simulink model "GaitAlgorithm_arduino_V3_2024a"  (R2024b)
settings: Solver=FixedStepAuto  StartTime=0.0  StopTime=inf  RelTol=1e-3  EnableMultiTasking=on
undefined symbols (not defined in the file): DiscIntNeverNeededParam, f
libraries: simulink x16, mcp2515lib x13, matrix_library x6, arduinosensorlib x4, eeGeneralControl x4, arduinolib x2, instrumentlib x2
(part 1 of 2)
settings Model: ExtModeTrigDuration=2  Creator=82108  LastModifiedBy=admin
settings SolverCC: AutoInsertRateTranBlk=on
settings OptimizationCC: EnhancedBackFolding=on  PassReuseOutputArgsAs=Individual arguments  ZeroExternalMemoryAtStartup=off  ZeroInternalMemoryAtStartup=off  MaxStackSize=64  OptimizeBlockOrder=speed  DifferentSizesBufferReuse=on  OptimizationCustomize=off  EfficientTunableParamExpr=on
settings DebuggingCC: ParameterTunabilityLossMsg=error
settings HardwareCC: ProdBitPerInt=16  ProdBitPerPointer=16  ProdBitPerSizeT=16  ProdBitPerPtrDiffT=16  ProdLargestAtomicFloat=None  ProdWordSize=8  ProdHWDeviceType=Atmel->AVR  TargetBitPerPointer=64  TargetBitPerSizeT=64  TargetBitPerPtrDiffT=64  TargetLongLongMode=on  TargetIntDivRoundTo=Zero  TargetEndianess=LittleEndian  TargetWordSize=64  TargetHWDeviceType=Custom Processor->MATLAB Host Computer  ProdEqTarget=off
settings SFSimCC: MATLABDynamicMemAlloc=off
settings RTWCC: Description=Embedded Coder  SystemTargetFile=ert.tlc  HardwareBoard=Arduino Uno  TemplateMakefile=ert_default_tmf  Toolchain=Arduino AVR  BuildConfiguration=Faster Runs  GPUComputeCapability=3.5
settings CodeAppCC: ForceParamTrailComments=on  IgnoreCustomStorageClasses=off  OperatorAnnotations=on  SimulinkDataObjDesc=on  SFDataObjDesc=on  InsertBlockDesc=on
settings ERTTargetCC: SupportContinuousTime=on  SupportVariableSizeSignals=on  ExtModeTransport=3  ExtModeStaticAlloc=on  ExtModeAutomaticAllocSize=off  ExtModeStaticAllocSize=250  ExtModeMexFile=ext_xcp  ExtModeIntrfLevel=Level2 - Open  InlinedParameterPlacement=Hierarchical  DynamicArrayContainerType=coder::array

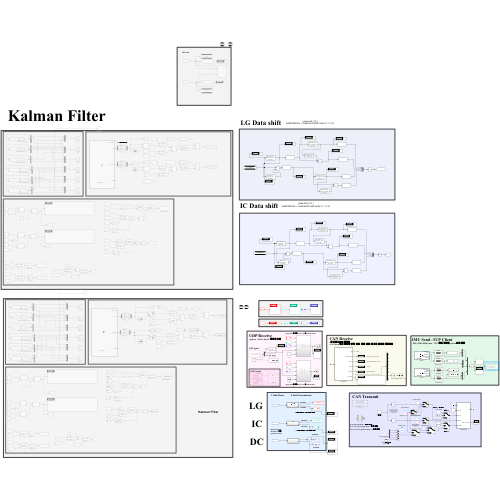
[thumbnail: Simulink's stored preview of the top-level diagram]
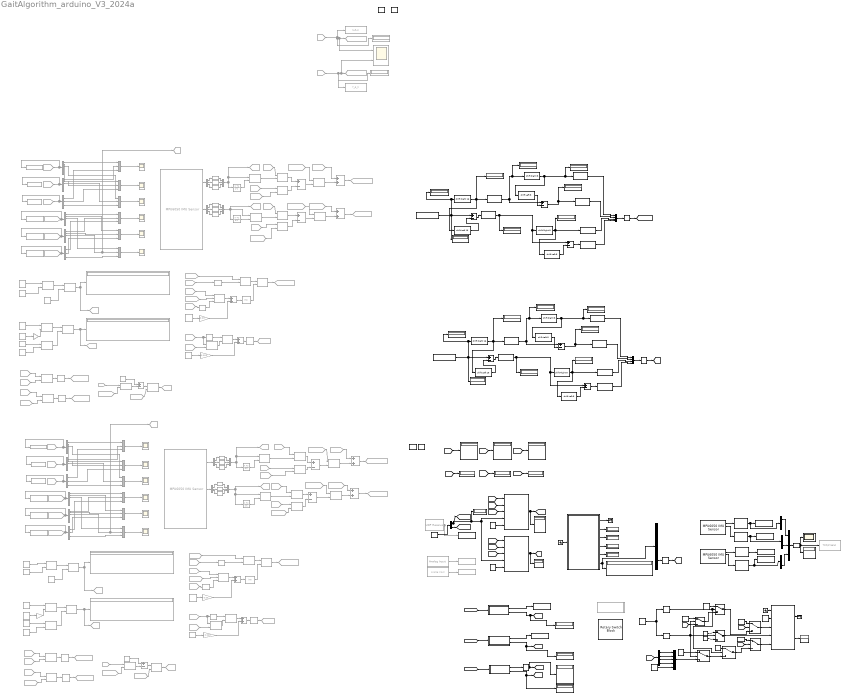
== system GaitAlgorithm_arduino_V3_2024a ==
  note: data 전달받았는지 확인
  note: gait phase에 따른 DC, IC, LG 의 position value
  note: LG Data shift
  note: [ data shift 과정 ]
      | 0xABCDEFGH -> 0xAB 0xCD 0xEF 0xGH 로 나눠줌
  note: position
  note: Kalman Filter
  note: IMU data
  note: Kalman Filter
  note: bias 로 영점 조절
  note: DC
  note: MobileNetHED- Double3D 기반
      | gait phase label
  note: 16진수 데이터 ID로 나눠서 전송
  note: id value
  note: Gait Phase
  note: 2. Data Transmission
  note: 16진수 데이터 ID로 나눠서 전송
  note: id value
  note: position
  note: LG
  note: IC
  note: position
  note: id value
  note: CAN Receive
      | :모터에 나오는 데이터
      | :CAN data에서 모터의 위치, 속도, 전류, 온도 등 모터 정보를 제공받음
  note: gait phase에 따른 DC, IC, LG 의 CAN id value
  note: UDP signal
  note: EMG signal
  note: extended version인지 확인
  note: id 확인
  note: data length 확인
  note: 온도 255 degree 넘으면 중지
  note: etc
  note: etc
  note: IC Data shift
  note: IMU Send -TCP Client
      | :IMU (MPU6050) data - TCP 통신 이용해 python으로 전달
  note: UDP Receive
      | :python - label1, label2 데이터 수신
  note: [ data shift 과정 ]
      | 0xABCDEFGH -> 0xAB 0xCD 0xEF 0xGH 로 나눠줌
  note: 모드
  note: motor position value
  note: D (0): Driving mode - 운용 모드
      | Z (1): Zeroing (origin) mode - 영점 조절
      | TZ (2): To Zero position mode - 0으로 복귀
  note: 틀리면 0 / 맞으면 1
      | - driving mode: 00
      | - zeroing mode: 01
      | - to zero: 10
  note: driving mode : id
  note: driving mode
      | & to zero mode : DLC
  note: 온도 limit
  note: to zero mode : data
  note: 온도 limit
  note: zeroing mode : DLC
  note: 온도가 limit 초과할 시,
      | to zero mode
  note: CAN Transmit
  note: to zero mode : id
  note: shape 맞추기 위한 dummy 값
  note: zeroing mode : id
  note: zeroing mode :
      | data
  Acc_x : Scope  Commented=on
  Acc_x1 : Scope  Commented=on
  Acc_y : Scope  Commented=on
  Acc_y1 : Scope  Commented=on
  Acc_z : Scope  Commented=on
  Acc_z1 : Scope  Commented=on
  Add{,1,6,9..10,13..15} (8 alike) : Sum  Commented=on
  Add{5,7..8,11..12,16} (6 alike) : Sum  Commented=on  Inputs=+-
  Add{2..4,17..19} (6 alike) : Sum  Inputs=+-
  Analog Input : arduinolib/Analog Input  Commented=on  pinNumber=0  ReadResultsOnly=off  ConversionTriggerSource=Software  ExternalTriggerType=uint32( 0 )  OutputDataType=uint16  EnableConversionCompleteNotify=off  EnableOuputStatus=off  SampleTime=0.01  blockPlatform=arduino
      settings: SourceProductName=Common
  Analog Input1 : arduinolib/Analog Input  Commented=on  pinNumber=1  ReadResultsOnly=off  ConversionTriggerSource=Software  ExternalTriggerType=uint32( 0 )  OutputDataType=uint16  EnableConversionCompleteNotify=off  EnableOuputStatus=off  SampleTime=0.01  blockPlatform=arduino
      settings: SourceProductName=Common
  Bias{,1..11} (12 alike) : Bias  Commented=on  SaturateOnIntegerOverflow=off
  CANbegin : Subsystem  Commented=on  TreatAsAtomicUnit=on  mask{TargetHardware=Arduino, Oscillator=8, CANSpeed=1000, CSpin=10}
      mask prompts: TargetHardware "Target Hardware"; Oscillator "Oscillator frequency(MHz)"; CANSpeed "CAN speed(kHz)"; CSpin "Chip Select Pin"
      mask init:
      | % Get this mask's handle
      | maskObj = Simulink.Mask.get(gcb);
      | 
      | % Get the selected value from mask parameter's option
      | str_TargetHard = char(maskObj.Parameters(1).TypeOptions(TargetHardware));
      | str_Osc = char(maskObj.Parameters(2).TypeOptions(Oscillator));
      | str_CANSpeed = char(maskObj.Parameters(3).TypeOptions(CANSpeed));
      | 
      | % Set Icon
      | str1 = sprintf('%s(Model)',str_TargetHard);
      | str2 = sprintf('Oscillator: %s(MHz)',str_Osc);
      | str3 = sprintf('CAN Bus Speed: %s(kHz)',str_CANSpeed);
      | str4 = sprintf('Chip Select pin: %d',CSpin);
      | 
      | % Set the values of Variant Subsystem
      | switch str_TargetHard
      |     case 'Arduino'
      |         str = [str1,'\n',str2,'\n',str3,'\n',str4];
      |         evalin('base',sprintf('CSpin = %d;',CSpin));        
      |         evalin('base','Hardware = 1;');
      |     case 'Raspberry Pi'
      |         str = [str1,'\n',str2,'\n',str3];
      |         evalin('base',sprintf('clear CSpin',CSpin));           
      |         evalin('base','Hardware = 2;');     
      | end  
      | 
      | % Get the CAN Configuration register's value from mask parameter's option
      | if str_Osc == '8' %[MHz]
      |     switch str_CANSpeed
      |         case '1000'
      |             BPR = 0; PHSEG1 = 0; PRSEG = 0; PHSEG2 = 0;
      |         case '500'
      |             BPR = 0; PHSEG1 = 2; PRSEG = 0; PHSEG2 = 2;
      |         case '250'
      |             BPR = 0; PHSEG1 = 6; PRSEG = 0; PHSEG2 = 6;
      |         case '125'
      |             BPR = 1; PHSEG1 = 6; PRSEG = 1; PHSEG2 = 5;
      |         case '100'
      |             BPR = 1; PHSEG1 = 7; PRSEG = 2; PHSEG2 = 7;
      |         case '83.3'
      |             BPR = 1; PHSEG1 = 7; PRSEG = 6; PHSEG2 = 7;
      |         case '62.5'
      |             BPR = 3; PHSEG1 = 6; PRSEG = 0; PHSEG2 = 6;
      |         case '50'
      |             BPR = 3; PHSEG1 = 7; PRSEG = 2; PHSEG2 = 7;
      |         case '33.3'
      |             BPR = 4; PHSEG1 = 7; PRSEG = 6; PHSEG2 = 7;
      |     end            
      | elseif str_Osc == '16' %[MHz]
      |     switch str_CANSpeed  
      |         case '1000'
      |             BPR = 0; PHSEG1 = 2; PRSEG = 0; PHSEG2 = 2;
      |         case '500'
      |             BPR = 0; PHSEG1 = 6; PRSEG = 0; PHSEG2 = 6;
      |         case '250'
      |             BPR = 1; PHSEG1 = 6; PRSEG = 1; PHSEG2 = 5;        
      |         case '125'
      |             BPR = 3; PHSEG1 = 6; PRSEG = 0; PHSEG2 = 6;
      |         case '100'
      |             BPR = 3; PHSEG1 = 7; PRSEG = 2; PHSEG2 = 7;
      |         case '83.3'
      |             BPR = 3; PHSEG1 = 7; PRSEG = 6; PHSEG2 = 7;
      |         case '62.5'
      |             BPR = 7; PHSEG1 = 6; PRSEG = 0; PHSEG2 = 6;
      |         case '50'
      |             BPR = 7; PHSEG1 = 7; PRSEG = 2; PHSEG2 = 7;
      |         case '33.3'
      |             BPR = 9; PHSEG1 = 7; PRSEG = 6; PHSEG2 = 7;        
      |     end   
      | end
      | % Set the CAN Configuration register's value
      | address2A = BPR;          % bit7-6 :SJW, bit5-0: BPR
      | address29 = 192 ...       % bit7: BTLMODE = 1, bit6:SAM = 1
      |             + 8*PHSEG1 ...% bit5-3: PHSEG1
      |             +PRSEG;       % bit2-0: PRSEG
      | address28 = 128 ...       % bit7: SOF = 1, bit6:WAKFIL = 0
      |             + PHSEG2;     % bit5-3: 0, bit2-0: PHSEG2
      settings: RTWSystemCode=Nonreusable function
      mask TypeOptions TargetHardware: Arduino | Raspberry Pi
      mask Callback TargetHardware:
      | if(strcmp(get_param(gcb,'TargetHardware'),'Arduino'))
      |     set_param(gcb,'MaskVisibilities',{'on','on','on','on'})
      | else
      |     set_param(gcb,'MaskVisibilities',{'on','on','on','off'})
      | end
      mask TypeOptions Oscillator: 8 | 16
      mask TypeOptions CANSpeed: 1000 | 500 | 250 | 125 | 100 | 83.3 | 62.5 | 50 | 33.3
      mask DialogControl DescGroupVar Prompt: Description
      mask DialogControl DescTextVar Prompt: This block must be executed only once when beginning CAN communication because MCP2515’s register needs to be configured. And the frequency of oscillator for MCP2515 is also needed because it effects to the setting parameters of MCP2515's register.
      mask Display: disp(str)
  CANreceive : Subsystem  TreatAsAtomicUnit=on
      mask DialogControl DescGroupVar Prompt: Description
      mask DialogControl DescTextVar Prompt: CANreceive outputs CAN data by converting MCP2515 RX buffer register’s values. In/Out ports are no use because they are used for controlling the execution order. CAN_Received outputs 1(CAN received) or -1( No message).
  CANtransmit : Subsystem  TreatAsAtomicUnit=on
      mask DialogControl DescGroupVar Prompt: Description
      mask DialogControl DescTextVar Prompt: CANtransmit inputs CAN data by converting MCP2515 TX buffer register’s values. In/Out ports are no use because they are used for controlling the execution order. CAN_Transmitted outputs 1(Success) or 2(Fail).
  Compare To Constant7 : simulink/Logic and Bit Operations/Compare To Constant  relop===  const=1  OutDataTypeStr=boolean
  Compare To Constant8 : simulink/Logic and Bit Operations/Compare To Constant  relop===  const=2  OutDataTypeStr=boolean
  Compare To Constant9 : simulink/Logic and Bit Operations/Compare To Constant  relop=>=  const=0xff  OutDataTypeStr=boolean
  Constant : Constant  Value=[0 0 0 0]  OutDataTypeStr=uint8
  Constant1 : Constant  OutDataTypeStr=uint8
  Constant10 : Constant  Commented=on  Value=[0 0 0; 0 0 0; 0 0 0]  SampleTime=-1
  Constant11 : Constant  Commented=on  Value=[0 0 0; 0 0 0; 0 0 0]
  Constant12 : Constant  Commented=on  Value=[0 0 0 0 0 0; 0 0 0 0 0 0; 0 0 0 0 0 0]
  Constant13 : Constant  Commented=on  Value=[0 0 0; 0 0 0; 0 0 0]
  Constant14 : Constant  Value=0x168  OutDataTypeStr=uint16
  Constant15 : Constant  Value=[0x00 0x00 0x07 0xd0 ]  OutDataTypeStr=uint16
  Constant2 : Constant  Value=[1,1]
  Constant21 : Constant  Value=0x468
  Constant22 : Constant  Value=[0 0 0 0 0 0 0 0 ]  OutDataTypeStr=uint8
  Constant23 : Constant  Value=0x468
  Constant24 : Constant  Value=[0 0 0 0 0 0 0 0 ]  OutDataTypeStr=uint8
  Constant25 : Constant
  Constant3 : Constant  Value=4  OutDataTypeStr=uint8
  Constant5 : Constant  Value=0x568
  Constant6 : Constant  OutDataTypeStr=uint8
  Constant7 : Constant  Value=[0x01 0 0 0 0 0 0 0]  OutDataTypeStr=uint8
  Constant8 : Constant  Commented=on  Value=[0 0 0; 0 0 0; 0 0 0]
  Constant9 : Constant  Commented=on  Value=[0 0 0 0 0 0; 0 0 0 0 0 0; 0 0 0 0 0 0]  SampleTime=-1
  Data Store Memory : DataStoreMemory  DataStoreName=T_G_Z  WriteAfterWriteMsg=warning  ShowAdditionalParam=off
  Data Store Memory1 : DataStoreMemory  DataStoreName=S_G_Z  WriteAfterWriteMsg=warning  ShowAdditionalParam=off
  Data Store Memory2 : DataStoreMemory  DataStoreName=LG_position  WriteAfterWriteMsg=warning  ShowAdditionalParam=off
  Data Store Memory4 : DataStoreMemory  DataStoreName=IC_position  WriteAfterWriteMsg=warning  ShowAdditionalParam=off
  Data Store Read : DataStoreRead  DataStoreName=LG_position  IndexOptions=Index vector (dialog)  Indices=1  OutputSizes=1
  Data Store Read3 : DataStoreRead  DataStoreName=IC_position  IndexOptions=Index vector (dialog)  Indices=1  OutputSizes=1
  Data Store Write : DataStoreWrite  Commented=on  DataStoreName=T_G_Z  DataStoreElements=T_G_Z  IndexOptions=Index vector (dialog)  Indices=1  OutputSizes=1
  Data Store Write1 : DataStoreWrite  Commented=on  DataStoreName=S_G_Z  DataStoreElements=S_G_Z  IndexOptions=Index vector (dialog)  Indices=1  OutputSizes=1
  Data Store Write2 : DataStoreWrite  DataStoreName=LG_position  IndexOptions=Index vector (dialog)  Indices=1  OutputSizes=1
  Data Store Write3 : DataStoreWrite  DataStoreName=IC_position  IndexOptions=Index vector (dialog)  Indices=1  OutputSizes=1
  Data Type Conversion{1..2,10..11} (4 alike) : DataTypeConversion  OutDataTypeStr=uint16  SaturateOnIntegerOverflow=off  RndMeth=Floor
  Data Type Conversion{6..7,9,12} (4 alike) : DataTypeConversion  OutDataTypeStr=uint8  SaturateOnIntegerOverflow=off  RndMeth=Floor
  Data Type Conversion{3..5,8} (4 alike) : DataTypeConversion  OutDataTypeStr=uint8  RndMeth=Floor
  Delay1 : Delay  Commented=on  DelayLength=1
  Delay2 : Delay  Commented=on  DelayLength=1
  Delay_acc : Delay  Commented=on  DelayLength=1  InitialCondition=[0; 0; 0; 0; 0;0]
  Delay_acc1 : Delay  Commented=on  DelayLength=1  InitialCondition=[0; 0; 0; 0; 0;0]
  Delay_gyro : Delay  Commented=on  DelayLength=1  InitialCondition=[0; 0; 0; 0; 0;0]
  Delay_gyro1 : Delay  Commented=on  DelayLength=1  InitialCondition=[0; 0; 0; 0; 0;0]
  Demux : Demux  Outputs=8
  Demux1 : Demux  Outputs=3
  Demux{3..4,6..7,9..10,16,18} (8 alike) : Demux  Commented=on  Outputs=6
  Demux{5,8,11..15,17} (8 alike) : Demux  Commented=on  Outputs=3
  Demux19 : Demux  Outputs=3
  Demux2 : Demux
  Demux20 : Demux  Outputs=3
  Demux22 : Demux  Outputs=2
  Discrete-Time Integrator{,1..3} (4 alike) : DiscreteIntegrator  Commented=on  SampleTime=-1  ICPrevOutput=DiscIntNeverNeededParam  ICPrevScaledInput=DiscIntNeverNeededParam
  Display{,1,7,9..41} (36 alike) : Display
      Display11 settings: Format=hex (Stored Integer)
      Display12 settings: Format=hex (Stored Integer)
      Display13 settings: Format=hex (Stored Integer)
      Display14 settings: Format=hex (Stored Integer)
      Display15 settings: Format=hex (Stored Integer)
      Display16 settings: Format=hex (Stored Integer)
      Display17 settings: Format=hex (Stored Integer)
      Display18 settings: Format=hex (Stored Integer)
      Display19 settings: Format=hex (Stored Integer)
      Display20 settings: Format=hex (Stored Integer)
      Display21 settings: Format=hex (Stored Integer)
      Display22 settings: Format=hex (Stored Integer)
      Display23 settings: Format=hex (Stored Integer)
      Display24 settings: Format=hex (Stored Integer)
      Display28 settings: Format=hex (Stored Integer)
      Display30 settings: Format=hex (Stored Integer)
      Display32 settings: Format=hex (Stored Integer)
      Display7 settings: Format=hex (Stored Integer)
  Display{2..6,8} (6 alike) : Display  Commented=on
  Enabled Subsystem1 : Subsystem  TreatAsAtomicUnit=on
  Enabled Subsystem3 : Subsystem  TreatAsAtomicUnit=on
  Enabled Subsystem4 : Subsystem  TreatAsAtomicUnit=on
  Estimated_Data_acc : From  Commented=on  GotoTag=x_hat
  Estimated_Data_acc1 : From  Commented=on  GotoTag=x_hat_2
  Estimated_Data_gyro : From  Commented=on  GotoTag=AR_x_hat
  Estimated_Data_gyro1 : From  Commented=on  GotoTag=AR_x_hat_2
  From1 : From  Commented=on  GotoTag=C_Phi
  From10 : From  Commented=on  GotoTag=AR_x_bar
  From12 : From  Commented=on  GotoTag=x_hat
  From{3,9,13,18,48..51} (8 alike) : From  Commented=on  GotoTag=H
  From14 : From  Commented=on  GotoTag=x_bar
  From15 : From  Commented=on  GotoTag=kalmangain
  From16 : From  Commented=on  GotoTag=x_bar
  From17 : From  Commented=on  GotoTag=kalmangain
  From19 : From  Commented=on  GotoTag=cov_bar
  From2 : From  Commented=on  GotoTag=cov
  From20 : From  Commented=on  GotoTag=C_Phi_2
  From21 : From  Commented=on  GotoTag=cov_2
  From22 : From  Commented=on  GotoTag=AR_x_bar_2
  From23 : From  Commented=on  GotoTag=kalmangain
  From24 : From  Commented=on  GotoTag=AR_x_bar
  From25 : From  Commented=on  GotoTag=C_Phi
  From26 : From  Commented=on  GotoTag=AR_x_hat
  From{27,29,34,43..47} (8 alike) : From  Commented=on  GotoTag=H_2
  From28 : From  Commented=on  GotoTag=x_hat_2
  From30 : From  Commented=on  GotoTag=x_bar_2
  From31 : From  Commented=on  GotoTag=kalmangain_2
  From32 : From  Commented=on  GotoTag=x_bar_2
  From33 : From  Commented=on  GotoTag=kalmangain_2
  From35 : From  Commented=on  GotoTag=cov_bar_2
  From36 : From  Commented=on  GotoTag=C_Phi_2
  From37 : From  Commented=on  GotoTag=kalmangain_2
  From38 : From  Commented=on  GotoTag=AR_x_bar_2
  From39 : From  Commented=on  GotoTag=C_Phi_2
  From4 : From  Commented=on  GotoTag=C_Phi
  From40 : From  Commented=on  GotoTag=AR_x_hat_2
  From41 : From  Commented=on  GotoTag=cov_bar_2
  From42 : From  Commented=on  GotoTag=cov_bar_2
  From5 : From  Commented=on  GotoTag=cov_bar
  From52 : From  Commented=on  GotoTag=TGZ
  From53 : From  Commented=on  GotoTag=SGZ
  From6 : From  Commented=on  GotoTag=cov_bar
  Gain : Gain  Commented=on  Gain=-0.01
  Gain1 : Gain  Commented=on  Gain=-0.01
  Goto : Goto  Commented=on  GotoTag=thigh_gyro_z
  Goto1 : Goto  Commented=on  GotoTag=C_Phi
  Goto10 : Goto  Commented=on  GotoTag=AR_x_bar
  Goto11 : Goto  Commented=on  GotoTag=x_hat_2
  Goto12 : Goto  Commented=on  GotoTag=AR_x_bar_2
  Goto13 : Goto  Commented=on  GotoTag=x_bar_2
  Goto14 : Goto  Commented=on  GotoTag=cov_bar_2
  Goto15 : Goto  Commented=on  GotoTag=H_2
  Goto16 : Goto  Commented=on  GotoTag=cov_2
  Goto17 : Goto  Commented=on  GotoTag=x_2
  Goto18 : Goto  Commented=on  GotoTag=AR_x_hat_2
  Goto19 : Goto  Commented=on  GotoTag=AR_x_2
  Goto2 : Goto  Commented=on  GotoTag=x_hat
  Goto20 : Goto  Commented=on  GotoTag=cov
  Goto21 : Goto  Commented=on  GotoTag=x
  Goto22 : Goto  Commented=on  GotoTag=AR_x_hat
  Goto23 : Goto  Commented=on  GotoTag=AR_x
  Goto24 : Goto  Commented=on  GotoTag=SGZ
  Goto25 : Goto  Commented=on  GotoTag=TGZ
  Goto4 : Goto  Commented=on  GotoTag=x_bar
  Goto6 : Goto  Commented=on  GotoTag=shank_gyro_z
  Goto7 : Goto  Commented=on  GotoTag=cov_bar
  Goto8 : Goto  Commented=on  GotoTag=C_Phi_2
  Goto9 : Goto  Commented=on  GotoTag=H
  Ground : Ground
  Ground1 : Ground
  Gyro_x : Scope  Commented=on
  Gyro_x1 : Scope  Commented=on
  Gyro_y : Scope  Commented=on
  Gyro_y1 : Scope  Commented=on
  Gyro_z : Scope  Commented=on
  Gyro_z1 : Scope  Commented=on
  IdentityMatrix{,1..2,4,7..9,11} (8 alike) : IdentityMatrix  Commented=on  OutputDimensions=3  SampleTime=-1
  IdentityMatrix{3,5..6,10,12..13} (6 alike) : IdentityMatrix  Commented=on  OutputDimensions=6  SampleTime=-1
  Kalman_Gain : Goto  Commented=on  GotoTag=kalmangain
  Kalman_Gain1 : Goto  Commented=on  GotoTag=kalmangain_2
  MPU6050 IMU Sensor : arduinosensorlib/MPU6050 IMU Sensor  Commented=on  I2CModule=0  SlaveAddress=0x68  Accel=on  AngularRate=on  Temperature=off  Status=on  Timestamp=off  EulerAngles=off  Quat=off  AccelRange=2G  GyroRange=250 dps  DmpOdr=200 Hz  Dlpf=Accelerometer: 184Hz, Gyroscope: 188Hz  spf=1  SampleTime=0.01  QueueSizeFactor=1
      settings: SourceProductName=Sensors
  MPU6050 IMU Sensor1 : arduinosensorlib/MPU6050 IMU Sensor  Commented=on  I2CModule=0  SlaveAddress=0x69  Accel=on  AngularRate=on  Temperature=off  Status=on  Timestamp=off  EulerAngles=off  Quat=off  AccelRange=2G  GyroRange=250 dps  DmpOdr=200 Hz  Dlpf=Accelerometer: 184Hz, Gyroscope: 188Hz  spf=1  SampleTime=0.01  QueueSizeFactor=1
      settings: SourceProductName=Sensors
  Matrix Concatenate{,1,4,7..8,11} (6 alike) : Concatenate  Commented=on  Mode=Multidimensional array  ConcatenateDimension=2
  Matrix Concatenate{2..3,5..6,9..10,12..13} (8 alike) : Concatenate  Commented=on  Mode=Multidimensional array
  Matrix Divide : Product  Commented=on  Inputs=/  Multiplication=Matrix(*)
  Matrix Divide1 : Product  Commented=on  Inputs=/  Multiplication=Matrix(*)
  Matrix Multiply{,1..3,5..23,25..29} (28 alike) : Product  Commented=on  Multiplication=Matrix(*)
  Matrix Multiply24 : Product  Commented=on  Inputs=3  Multiplication=Matrix(*)
  Matrix Multiply4 : Product  Commented=on  Inputs=3  Multiplication=Matrix(*)
  Measurement_Data_acc : From  Commented=on  GotoTag=x
  Measurement_Data_acc1 : From  Commented=on  GotoTag=x_2
  Measurement_Data_gyro : From  Commented=on  GotoTag=AR_x
  Measurement_Data_gyro1 : From  Commented=on  GotoTag=AR_x_2
  Mux{,1..15} (16 alike) : Mux  Commented=on  Inputs=3
  Mux16 : Mux  Inputs=3
  Predicted_Data_acc : From  Commented=on  GotoTag=x_bar
  Predicted_Data_acc1 : From  Commented=on  GotoTag=x_bar_2
  Predicted_Data_gyro : From  Commented=on  GotoTag=AR_x_bar
  Predicted_Data_gyro1 : From  Commented=on  GotoTag=AR_x_bar_2
  Reshape1 : Reshape
  Reshape2 : Reshape
  Reshape3 : Reshape
  Reshape4 : Reshape  OutputDimensionality=Customize  OutputDimensions=[3,1]
  Rotary Switch : RotarySwitchBlock
      settings: Values={{'D', 'Z', 'TZ'}, [0 1 2]}
  Scope1 : Scope  Commented=on  NumInputPorts=2
  Scope2 : Scope
  Shift Arithmetic{1,7,10..11} (4 alike) : ArithShift  BitShiftNumber=8  BitShiftDirection=Right
  Shift Arithmetic13 : ArithShift  BitShiftNumber=16  BitShiftDirection=Right
  Shift Arithmetic{2,4,6,9} (4 alike) : ArithShift  BitShiftNumber=8  BitShiftDirection=Left
  Shift Arithmetic3 : ArithShift  BitShiftNumber=16  BitShiftDirection=Left
  Shift Arithmetic5 : ArithShift  BitShiftNumber=16  BitShiftDirection=Right
  Shift Arithmetic8 : ArithShift  BitShiftNumber=16  BitShiftDirection=Left
  Subsystem : Subsystem
  Subsystem1 : Subsystem
  Switch{,1..4,11..12} (7 alike) : Switch  Criteria=u2 > Threshold  SaturateOnIntegerOverflow=off  InputSameDT=off
  TCP/IP Send2 : instrumentlib/TCP//IP Send  Commented=on  Host=172.16.1.77  Port=5550  ByteOrder=little-endian  EnableBlockingMode=on  Timeout=10  TransferDelay=off  SimulateUsing=Interpreted execution
  Terminator : Terminator
  Terminator1 : Terminator
  To Workspace : ToWorkspace  Commented=on  VariableName=predicted_acc  SaveFormat=Timeseries  SampleTime=-1
  To Workspace1 : ToWorkspace  Commented=on  VariableName=measured_acc  SaveFormat=Timeseries  SampleTime=-1
  To Workspace10 : ToWorkspace  Commented=on  VariableName=estimated_gyro_shank  SaveFormat=Timeseries  SampleTime=-1
  To Workspace11 : ToWorkspace  Commented=on  VariableName=measured_gyro_shank  SaveFormat=Timeseries  SampleTime=-1
  To Workspace12 : ToWorkspace  VariableName=predicted  SaveFormat=Timeseries  SampleTime=-1
  To Workspace13 : ToWorkspace  Commented=on  VariableName=emg0  SaveFormat=Timeseries  SampleTime=-1
  To Workspace14 : ToWorkspace  Commented=on  VariableName=emg1  SaveFormat=Timeseries  SampleTime=-1
  To Workspace15 : ToWorkspace  VariableName=shank_acc  SaveFormat=Timeseries  SampleTime=0.01
  To Workspace16 : ToWorkspace  VariableName=shank_gyro  SaveFormat=Timeseries  SampleTime=0.01
  To Workspace17 : ToWorkspace  VariableName=thigh_acc  SaveFormat=Timeseries  SampleTime=-1
  To Workspace18 : ToWorkspace  VariableName=thigh_gyro  SaveFormat=Timeseries  SampleTime=-1
  To Workspace2 : ToWorkspace  Commented=on  VariableName=estimated_acc  SaveFormat=Timeseries  SampleTime=-1
  To Workspace3 : ToWorkspace  Commented=on  VariableName=predicted_gyro  SaveFormat=Timeseries  SampleTime=-1
  To Workspace4 : ToWorkspace  Commented=on  VariableName=estimated_gyro  SaveFormat=Timeseries  SampleTime=-1
  To Workspace5 : ToWorkspace  Commented=on  VariableName=measured_gyro  SaveFormat=Timeseries  SampleTime=-1
  To Workspace6 : ToWorkspace  Commented=on  VariableName=predicted_acc_shank  SaveFormat=Timeseries  SampleTime=-1
  To Workspace7 : ToWorkspace  Commented=on  VariableName=measured_acc_shank  SaveFormat=Timeseries  SampleTime=-1
  To Workspace8 : ToWorkspace  Commented=on  VariableName=estimated_acc_shank  SaveFormat=Timeseries  SampleTime=-1
  To Workspace9 : ToWorkspace  Commented=on  VariableName=predicted_gyro_shank  SaveFormat=Timeseries  SampleTime=-1
  Transpose{,1..5} (6 alike) : matrix_library/Transpose  Commented=on
  UDP Receive : instrumentlib/UDP Receive  Commented=on  LocalAddress=172.16.1.77  LocalPort=8888  EnablePortSharing=off  Host=localhost  Port=9090  GetLatestData=off  DataSize=[ 2, 1 ]  DataType=uint8  ASCIIFormatting=%f,  Terminator=LF  CustomTerminator=10  ByteOrder=big-endian  EnableBlockingMode=on  Timeout=10  SampleTime=0.1  SimulateUsing=Interpreted execution
  Vector Concatenate1 : Concatenate  NumInputs=4  ConcatenateDimension=2
  Vector Concatenate2 : Concatenate  NumInputs=4  ConcatenateDimension=2
  Vector Concatenate3 : Concatenate  NumInputs=5
  sensor noise : Gain  Commented=on  Gain=0.03
  sensor noise1 : Gain  Commented=on  Gain=0.03
  shank1 : arduinosensorlib/MPU6050 IMU Sensor  I2CModule=0  SlaveAddress=0x68  Accel=on  AngularRate=on  Temperature=on  Status=on  Timestamp=off  EulerAngles=off  Quat=off  AccelRange=2G  GyroRange=250 dps  DmpOdr=200 Hz  Dlpf=Accelerometer: 184Hz, Gyroscope: 188Hz  spf=1  SampleTime=0.01  QueueSizeFactor=1
      settings: SourceProductName=Sensors
  shank_acc1 : eeGeneralControl/Low-Pass Filter (Discrete or Continuous)  K=1  T=0.029  B=inf  A=-inf  init_option=Inherited from block input  x0=0  Ts=0.01
  shank_gyro1 : eeGeneralControl/Low-Pass Filter (Discrete or Continuous)  K=1  T=0.029  B=inf  A=-inf  init_option=Inherited from block input  x0=0  Ts=-1
  system noise : Gain  Commented=on  Gain=0.005
  system noise1 : Gain  Commented=on  Gain=0.005
  thigh1 : arduinosensorlib/MPU6050 IMU Sensor  I2CModule=0  SlaveAddress=0x69  Accel=on  AngularRate=on  Temperature=on  Status=on  Timestamp=off  EulerAngles=off  Quat=off  AccelRange=2G  GyroRange=250 dps  DmpOdr=200 Hz  Dlpf=Accelerometer: 184Hz, Gyroscope: 188Hz  spf=1  SampleTime=0.01  QueueSizeFactor=1
      settings: SourceProductName=Sensors
  thigh_acc1 : eeGeneralControl/Low-Pass Filter (Discrete or Continuous)  K=1  T=0.029  B=inf  A=-inf  init_option=Inherited from block input  x0=0  Ts=-1
  thigh_gyro1 : eeGeneralControl/Low-Pass Filter (Discrete or Continuous)  K=1  T=0.029  B=inf  A=-inf  init_option=Inherited from block input  x0=0  Ts=-1
  wires:
  From52/1 -> Data Store Write/1, Display3/1, Scope1/2, Goto/1
  From53/1 -> Display2/1, Scope1/1, Goto6/1, Data Store Write1/1
  Add16/1 -> Matrix Multiply28/2
  Mux3/1 -> Gyro_x/1
  From24/1 -> Add9/1
  From10/1 -> Matrix Multiply12/2
  Demux6/2 -> Mux4/1
  Demux8/2 -> Mux4/3
  Demux7/3 -> Goto24/1, Mux5/2
  Measurement_Data_gyro/1 -> To Workspace5/1, Demux8/1
  Matrix Multiply13/1 -> Add9/2
  Transpose3/1 -> Matrix Multiply22/1
  From23/1 -> Matrix Multiply13/1
  Demux5/3 -> Mux2/3
  Estimated_Data_acc/1 -> To Workspace2/1, Demux4/1
  Demux3/3 -> Mux2/1
  Matrix Multiply11/1 -> Add8/1
  Demux5/2 -> Mux1/3
  Matrix Multiply9/1 -> Add7/2
  Add1/1 -> Matrix Divide/1
  Transpose2/1 -> Matrix Multiply4/3
  Matrix Multiply3/1 -> Matrix Multiply5/1
  From9/1 -> Transpose1/1
  From3/1 -> Matrix Multiply/1
  From13/1 -> Matrix Multiply7/1
  From12/1 -> Matrix Multiply6/2
  Transpose1/1 -> Matrix Multiply3/2
  Matrix Divide/1 -> Matrix Multiply5/2
  From5/1 -> Matrix Multiply3/1
  Delay_acc/1 -> Goto4/1
  Matrix Multiply5/1 -> Kalman_Gain/1
  Matrix Concatenate1/1 -> Matrix Concatenate2/2
  From48/1 -> Transpose2/1
  IdentityMatrix3/1 -> system noise/1
  Gain/1 -> Matrix Concatenate/2
  Matrix Concatenate4/1 -> Matrix Concatenate6/1
  From2/1 -> Matrix Multiply1/2
  Constant10/1 -> Matrix Concatenate4/2
  Delay1/1 -> Goto7/1
  Matrix Concatenate3/1 -> Matrix Multiply/2
  From4/1 -> Matrix Multiply1/1, Transpose/1
  Predicted_Data_acc/1 -> Demux3/1, To Workspace/1
  Matrix Concatenate2/1 -> Goto1/1, Display5/1
  Predicted_Data_gyro/1 -> To Workspace3/1, Demux6/1
  Matrix Concatenate6/1 -> Goto9/1, Display4/1
  Mux7/1 -> Acc_y1/1
  system noise/1 -> Add/2
  Demux8/3 -> Mux5/3
  system noise1/1 -> Add14/2
  From25/1 -> Matrix Multiply14/1
  Mux/1 -> Acc_x/1
  From46/1 -> Matrix Multiply18/1
  Constant9/1 -> Matrix Concatenate6/2
  Mux2/1 -> Acc_z/1
  Demux11/1 -> Mux9/3
  Matrix Multiply4/1 -> Add1/1
  Estimated_Data_acc1/1 -> To Workspace8/1, Demux16/1
  Demux4/2 -> Mux1/2
  Bias7/1 -> Mux14/1
  From50/1 -> Matrix Multiply11/1
  From43/1 -> Transpose4/1
  Matrix Concatenate10/1 -> Matrix Multiply15/2
  IdentityMatrix2/1 -> Matrix Concatenate1/2
  Matrix Multiply26/1 -> Delay_acc1/1
  From42/1 -> Matrix Multiply24/2
  Mux4/1 -> Gyro_y/1
  MPU6050 IMU Sensor1/1 -> Demux13/1  "x_now"
  From41/1 -> Matrix Multiply23/1
  sensor noise/1 -> Add1/2
  Mux15/1 -> Matrix Concatenate12/1, Discrete-Time Integrator3/1, Goto19/1
  Matrix Multiply8/1 -> Add6/2
  Matrix Multiply15/1 -> Add16/1
  Discrete-Time Integrator1/1 -> Matrix Concatenate5/2
  Demux9/2 -> Mux7/1
  From14/1 -> Matrix Multiply7/2
  Mux8/1 -> Acc_z1/1
  From1/1 -> Matrix Multiply6/1
  Demux10/1 -> Mux9/2
  Predicted_Data_acc1/1 -> Demux9/1, To Workspace6/1
  Demux6/1 -> Mux3/1
  IdentityMatrix1/1 -> Gain/1
  Matrix Multiply22/1 -> Add14/1
  Estimated_Data_gyro/1 -> To Workspace4/1, Demux7/1
  Bias9/1 -> Mux15/2
  Demux4/1 -> Mux/2
  Transpose4/1 -> Matrix Multiply23/2
  Bias10/1 -> Mux15/1
  Demux15/2 -> Bias9/1
  Demux8/1 -> Mux3/3
  Mux6/1 -> Acc_x1/1
  Bias11/1 -> Mux15/3
  Add13/1 -> Goto18/1
  Demux6/3 -> Mux5/1
  Delay2/1 -> Goto14/1
  Demux18/2 -> Mux10/1
  Bias8/1 -> Mux14/3
  Matrix Multiply24/1 -> Add15/1
  From26/1 -> Matrix Multiply14/2
  Mux13/1 -> Goto17/1, Matrix Concatenate10/1, Discrete-Time Integrator2/1
  IdentityMatrix11/1 -> Matrix Concatenate11/1
  From6/1 -> Matrix Multiply4/2
  Demux15/1 -> Bias10/1
  IdentityMatrix9/1 -> Matrix Concatenate8/2
  Demux14/1 -> Bias7/1
  Matrix Multiply20/1 -> Add13/2
  Mux1/1 -> Acc_y/1
  Demux3/2 -> Mux1/1
  Demux13/2 -> Bias3/1
  Bias6/1 -> Mux14/2
  Demux14/2 -> Bias6/1
  IdentityMatrix/1 -> Matrix Concatenate/1
  Demux4/3 -> Mux2/2
  Matrix Multiply6/1 -> Delay_acc/1
  From17/1 -> Matrix Multiply9/2
  Bias5/1 -> Mux13/3
  Bias3/1 -> Mux13/2
  Add5/1 -> Matrix Multiply8/2
  Bias2/1 -> Mux12/3
  Add7/1 -> Matrix Multiply10/1
  Constant8/1 -> Matrix Concatenate1/1
  Demux12/3 -> Bias2/1
  Demux12/1 -> Bias1/1
  Demux13/3 -> Bias5/1
  Add12/1 -> Matrix Multiply20/2
  From40/1 -> Matrix Multiply21/2
  Bias4/1 -> Mux13/1
  IdentityMatrix6/1 -> Add7/1
  Discrete-Time Integrator2/1 -> Matrix Concatenate10/2
  Bias1/1 -> Mux12/1
  From15/1 -> Matrix Multiply8/1
  MPU6050 IMU Sensor/1 -> Demux12/1  "x_now"
  Add8/1 -> Matrix Multiply13/2
  From37/1 -> Matrix Multiply20/1
  Add6/1 -> Goto2/1
  Matrix Multiply2/1 -> Add/1
  Demux14/3 -> Bias8/1
  Matrix Divide1/1 -> Matrix Multiply25/2
  Demux9/3 -> Mux8/1
  Matrix Multiply16/1 -> Matrix Multiply22/2
  Measurement_Data_gyro1/1 -> To Workspace11/1, Demux11/1
  Demux17/1 -> Mux6/3
  Measurement_Data_acc1/1 -> To Workspace7/1, Demux17/1
  Mux14/1 -> Matrix Concatenate5/1, Goto23/1, Discrete-Time Integrator1/1
  Demux9/1 -> Mux6/1
  Matrix Concatenate11/1 -> Matrix Concatenate13/1
  sensor noise1/1 -> Add15/2
  Demux7/2 -> Mux4/2
  Demux12/2 -> Bias/1
  Matrix Multiply19/1 -> Add12/2
  From16/1 -> Add6/1
  Matrix Multiply27/1 -> Add16/2
  From21/1 -> Matrix Multiply16/2
  Matrix Multiply12/1 -> Add8/2
  Bias/1 -> Mux12/2
  Matrix Multiply18/1 -> Add12/1
  Matrix Multiply21/1 -> Delay_gyro1/1
  From34/1 -> Matrix Multiply29/1
  Delay_gyro1/1 -> Goto12/1
  Demux16/3 -> Mux8/2
  Add14/1 -> Delay2/1
  Transpose5/1 -> Matrix Multiply24/3
  From29/1 -> Matrix Multiply27/1
  Demux15/3 -> Bias11/1
  From28/1 -> Matrix Multiply26/2
  Matrix Multiply25/1 -> Kalman_Gain1/1
  Matrix Multiply23/1 -> Matrix Multiply25/1
  From35/1 -> Matrix Multiply17/2
  From51/1 -> Matrix Multiply12/1
  From20/1 -> Matrix Multiply26/1
  From36/1 -> Matrix Multiply16/1, Transpose3/1
  IdentityMatrix13/1 -> Add11/1
  From47/1 -> Matrix Multiply19/1
  Constant11/1 -> Matrix Concatenate8/1
  MPU6050 IMU Sensor1/2 -> Demux15/1  "x_now_AR"
  Add/1 -> Delay1/1
  Delay_gyro/1 -> Goto10/1
  Demux18/1 -> Mux9/1
  Mux11/1 -> Gyro_z1/1
  Discrete-Time Integrator3/1 -> Matrix Concatenate12/2
  Demux13/1 -> Bias4/1
  From22/1 -> Matrix Multiply19/2
  Predicted_Data_gyro1/1 -> To Workspace9/1, Demux18/1
  Estimated_Data_gyro1/1 -> To Workspace10/1, Demux10/1
  IdentityMatrix12/1 -> sensor noise1/1
  Mux12/1 -> Goto21/1, Matrix Concatenate3/1, Discrete-Time Integrator/1
  Discrete-Time Integrator/1 -> Matrix Concatenate3/2
  Demux10/2 -> Mux10/2
  From38/1 -> Add13/1
  Demux18/3 -> Mux11/1
  Matrix Concatenate13/1 -> Goto15/1, Display6/1
  Matrix Concatenate/1 -> Matrix Concatenate2/1
  Demux7/1 -> Mux3/2
  Mux10/1 -> Gyro_y1/1
  From33/1 -> Matrix Multiply29/2
  IdentityMatrix4/1 -> Matrix Concatenate4/1
  From32/1 -> Add10/1
  IdentityMatrix10/1 -> system noise1/1
  From18/1 -> Matrix Multiply9/1
  Mux5/1 -> Gyro_z/1
  IdentityMatrix7/1 -> Matrix Concatenate7/1
  Matrix Concatenate5/1 -> Matrix Multiply11/2
  Matrix Concatenate7/1 -> Matrix Concatenate9/1
  Matrix Multiply1/1 -> Matrix Multiply2/2
  Demux10/3 -> Goto25/1, Mux11/2
  Matrix Multiply14/1 -> Delay_gyro/1
  Gain1/1 -> Matrix Concatenate7/2
  Demux3/1 -> Mux/1
  Matrix Concatenate12/1 -> Matrix Multiply18/2
  From49/1 -> Matrix Multiply4/1
  Matrix Concatenate8/1 -> Matrix Concatenate9/2
  Delay_acc1/1 -> Goto13/1
  Mux9/1 -> Gyro_x1/1
  From31/1 -> Matrix Multiply28/1
  Add11/1 -> Matrix Multiply17/1
  IdentityMatrix5/1 -> sensor noise/1
  Add9/1 -> Goto22/1
  Demux17/2 -> Mux7/3
  From19/1 -> Matrix Multiply10/2
  From39/1 -> Matrix Multiply21/1
  Add15/1 -> Matrix Divide1/1
  Add10/1 -> Goto11/1
  Demux17/3 -> Mux8/3
  Demux11/3 -> Mux11/3
  Measurement_Data_acc/1 -> To Workspace1/1, Demux5/1
  From45/1 -> Matrix Multiply24/1
  Constant13/1 -> Matrix Concatenate11/2
  IdentityMatrix8/1 -> Gain1/1
  Matrix Multiply29/1 -> Add11/2
  From30/1 -> Matrix Multiply27/2
  Matrix Multiply7/1 -> Add5/2
  Matrix Multiply/1 -> Add5/1
  From44/1 -> Transpose5/1
  Demux16/1 -> Mux6/2
  Matrix Multiply17/1 -> Goto16/1
  Constant12/1 -> Matrix Concatenate13/2
  Demux11/2 -> Mux10/3
  Demux16/2 -> Mux7/2
  Demux5/1 -> Mux/3
  MPU6050 IMU Sensor/2 -> Demux14/1  "x_now_AR"
  Matrix Concatenate9/1 -> Goto8/1, Display8/1
  Matrix Multiply10/1 -> Goto20/1
  From27/1 -> Matrix Multiply15/1
  Transpose/1 -> Matrix Multiply2/1
  Matrix Multiply28/1 -> Add10/2
  CANreceive/1(Out) -> Terminator1/1
  Ground1/1 -> CANreceive/1(In)
  CANreceive/2(CAN_Received) -> Display27/1
  CANreceive/3(CAN_ext) -> Display29/1
  CANreceive/4(CAN_id) -> Display30/1
  CANreceive/5(CAN_dlc) -> Display31/1
  CANreceive/6(CAN_data) -> Demux/1, Display32/1
  Enabled Subsystem4/2(Out2) -> Display33/1, [IC_id]
  Enabled Subsystem4/1(Out1) -> Data Store Write3/1
  Enabled Subsystem3/1(Out1) -> Reshape3/1
  Enabled Subsystem3/2(Out2) -> Display34/1, [DC_id]
  [pos_IC] -> Subsystem/2(In2)
  [IC_id] -> Subsystem1/2(In2)
  Constant15/1 -> Subsystem/5(In6)
  Constant14/1 -> Subsystem1/5(In6)
  Subsystem/1(Out1) -> Display10/1, [pos]
  Subsystem1/1(Out1) -> Display25/1, [id]
  Reshape3/1 -> Display35/1, [pos_DC]
  Enabled Subsystem1/2(Out2) -> Display26/1, [LG_id]
  Enabled Subsystem1/1(Out1) -> Data Store Write2/1
  Demux/7 -> Compare To Constant9/1
  Compare To Constant9/1 -> [temp]
  Analog Input/1 -> To Workspace13/1
  Analog Input1/1 -> To Workspace14/1
  Vector Concatenate1/1 -> Reshape1/1
  Shift Arithmetic10/1 -> Shift Arithmetic9/1, Display16/1, Data Type Conversion8/1
  Add17/1 -> Data Type Conversion3/1, Display15/1
  Shift Arithmetic8/1 -> Add18/2
  Data Type Conversion2/1 -> Display12/1, Add19/1, Shift Arithmetic10/1
  Shift Arithmetic6/1 -> Add17/2
  Data Type Conversion12/1 -> Vector Concatenate1/1
  Add18/1 -> Data Type Conversion2/1
  Data Type Conversion1/1 -> Add17/1, Display14/1, Shift Arithmetic1/1
  Data Type Conversion8/1 -> Vector Concatenate1/3
  Shift Arithmetic9/1 -> Add19/2
  Shift Arithmetic1/1 -> Shift Arithmetic6/1, Display11/1, Data Type Conversion12/1
  Data Type Conversion9/1 -> Vector Concatenate1/4
  Shift Arithmetic5/1 -> Shift Arithmetic8/1, Display24/1, Data Type Conversion1/1
  Add19/1 -> Data Type Conversion9/1
  Data Store Read/1 -> Add18/1, Display17/1, Display13/1, Shift Arithmetic5/1
  Reshape1/1 -> [pos_LG]
  Data Type Conversion3/1 -> Vector Concatenate1/2
  Shift Arithmetic13/1 -> Shift Arithmetic3/1, Display7/1, Data Type Conversion10/1
  Add4/1 -> Data Type Conversion6/1
  Data Type Conversion4/1 -> Vector Concatenate2/2
  Shift Arithmetic2/1 -> Add2/2
  Data Type Conversion5/1 -> Vector Concatenate2/3
  Shift Arithmetic3/1 -> Add3/2
  Reshape2/1 -> [pos_IC]
  Shift Arithmetic11/1 -> Shift Arithmetic2/1, Display18/1, Data Type Conversion7/1
  Vector Concatenate2/1 -> Reshape2/1
  Data Store Read3/1 -> Add3/1, Display28/1, Display20/1, Shift Arithmetic13/1
  Add2/1 -> Data Type Conversion4/1, Display22/1
  Data Type Conversion6/1 -> Vector Concatenate2/4
  Add3/1 -> Data Type Conversion11/1
  Data Type Conversion11/1 -> Display19/1, Add4/1, Shift Arithmetic7/1
  Shift Arithmetic4/1 -> Add4/2
  Data Type Conversion7/1 -> Vector Concatenate2/1
  Data Type Conversion10/1 -> Add2/1, Display21/1, Shift Arithmetic11/1
  Shift Arithmetic7/1 -> Shift Arithmetic4/1, Display23/1, Data Type Conversion5/1
  Demux20/3 -> Mux16/3
  shank1/2 -> shank_gyro1/1
  shank_acc1/1 -> To Workspace15/1, Demux1/1
  Demux1/1 -> Mux16/1
  thigh_gyro1/1 -> To Workspace18/1, Demux20/1
  Demux19/3 -> Mux16/2
  Mux16/1 -> Reshape4/1
  thigh_acc1/1 -> To Workspace17/1
  shank_gyro1/1 -> To Workspace16/1, Demux19/1
  thigh1/1 -> thigh_acc1/1
  thigh1/2 -> thigh_gyro1/1
  shank1/1 -> shank_acc1/1
  Reshape4/1 -> Scope2/1, Display9/1, TCP/IP Send2/1
  UDP Receive/1 -> To Workspace12/1
  [gait_phase] -> Enabled Subsystem1/1(In1)
  [gait_phase] -> Enabled Subsystem4/1(In1)
  [gait_phase] -> Enabled Subsystem3/1(In1)
  [id] -> Switch/3
  Constant25/1 -> Compare To Constant7/1, Compare To Constant8/1
  Constant3/1 -> Switch1/3
  Constant23/1 -> Switch11/1
  Switch4/1 -> Switch12/3
  Constant21/1 -> Switch3/1
  Constant24/1 -> Switch12/1
  Demux2/3 -> Vector Concatenate3/3
  CANtransmit/1(Out) -> Terminator/1
  [temp] -> Switch12/2
  Constant22/1 -> Switch4/1
  Switch11/1 -> CANtransmit/3(CAN_id)
  Demux2/4 -> Vector Concatenate3/4
  Vector Concatenate3/1 -> Switch2/3
  Ground/1 -> CANtransmit/1(In)
  Demux2/1 -> Vector Concatenate3/1
  Constant1/1 -> CANtransmit/2(CAN_ext)
  Constant5/1 -> Switch/1
  Compare To Constant7/1 -> Switch2/2, Switch1/2, Switch/2
  [pos] -> Demux2/1
  Compare To Constant8/1 -> Switch3/2, Switch4/2
  Switch2/1 -> Switch4/3
  Constant7/1 -> Switch2/1
  [temp] -> Switch11/2
  Constant6/1 -> Switch1/1
  Switch1/1 -> CANtransmit/4(CAN_dlc)
  CANtransmit/2(CAN_Transmitted) -> Display1/1
  Demux2/2 -> Vector Concatenate3/2
  Switch12/1 -> CANtransmit/5(CAN_data)
  Constant/1 -> Vector Concatenate3/5
  Switch/1 -> Switch3/3
  Switch3/1 -> Switch11/3
  Demux22/2 -> [gait_phase]
  Demux22/1 -> Display/1, Subsystem1/4(In5), Subsystem/4(In5), [gait_env]
  [pos_LG] -> Subsystem/1(In1)
  [pos_DC] -> Subsystem/3(In3)
  [DC_id] -> Subsystem1/3(In3)
  [LG_id] -> Subsystem1/1(In1)
  [pos_LG] -> Display36/1
  [pos_IC] -> Display37/1
  [pos_DC] -> Display38/1
  [DC_id] -> Display41/1
  [IC_id] -> Display40/1
  [LG_id] -> Display39/1
  Constant2/1 -> Demux22/1

== system GaitAlgorithm_arduino_V3_2024a/CANbegin ==
  Constant : Constant  Value=0  OutDataTypeStr=boolean  SampleTime=-1
  Temporary buffer : DataStoreMemory  DataStoreName=temp_1byte  ReadBeforeWriteMsg=warning  WriteAfterWriteMsg=warning  WriteAfterReadMsg=warning  ShowAdditionalParam=off  OutDataTypeStr=uint8
  Unit Delay : UnitDelay  InitialCondition=1  SampleTime=-1  HasFrameUpgradeWarning=on
  setup : Subsystem  TreatAsAtomicUnit=on
      settings: RTWSystemCode=Nonreusable function  RTWFileNameOpts=Use subsystem name
  wires:
  Unit Delay/1 -> setup/Enable
  Constant/1 -> Unit Delay/1

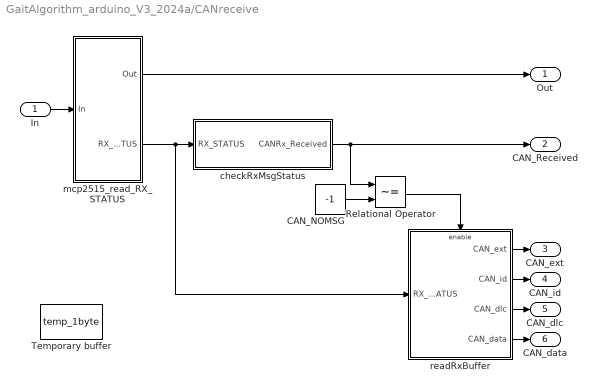
== system GaitAlgorithm_arduino_V3_2024a/CANreceive ==
  In : Inport
  CAN_NOMSG : Constant  Value=-1  OutDataTypeStr=int8
  Relational Operator : RelationalOperator  Operator=~=  OutDataTypeStr=boolean  InputSameDT=off
  Temporary buffer : DataStoreMemory  DataStoreName=temp_1byte  ReadBeforeWriteMsg=warning  WriteAfterWriteMsg=warning  WriteAfterReadMsg=warning  ShowAdditionalParam=off  OutDataTypeStr=uint8
  checkRxMsgStatus : Subsystem  TreatAsAtomicUnit=on
  mcp2515_read_RX_STATUS : Subsystem  TreatAsAtomicUnit=on
  readRxBuffer : Subsystem  TreatAsAtomicUnit=on
  Out : Outport
  CAN_Received : Outport  Port=2
  CAN_ext : Outport  Port=3
  CAN_id : Outport  Port=4
  CAN_dlc : Outport  Port=5
  CAN_data : Outport  Port=6
  wires:
  In/1 -> mcp2515_read_RX_STATUS/1(In)
  mcp2515_read_RX_STATUS/1(Out) -> Out/1
  checkRxMsgStatus/1(CANRx_Received) -> CAN_Received/1, Relational Operator/1
  mcp2515_read_RX_STATUS/2(RX_STATUS) -> readRxBuffer/1(RX_STATUS), checkRxMsgStatus/1(RX_STATUS)
  readRxBuffer/1(CAN_ext) -> CAN_ext/1
  readRxBuffer/2(CAN_id) -> CAN_id/1
  readRxBuffer/3(CAN_dlc) -> CAN_dlc/1
  readRxBuffer/4(CAN_data) -> CAN_data/1
  CAN_NOMSG/1 -> Relational Operator/2
  Relational Operator/1 -> readRxBuffer/Enable

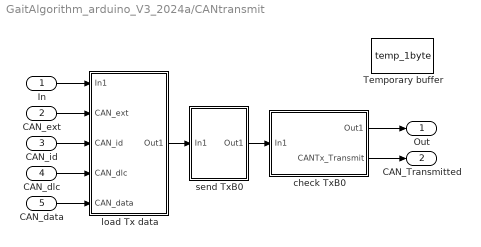
== system GaitAlgorithm_arduino_V3_2024a/CANtransmit ==
  In : Inport
  CAN_ext : Inport  Port=2
  CAN_id : Inport  Port=3
  CAN_dlc : Inport  Port=4
  CAN_data : Inport  Port=5
  Temporary buffer : DataStoreMemory  DataStoreName=temp_1byte  ReadBeforeWriteMsg=warning  WriteAfterWriteMsg=warning  WriteAfterReadMsg=warning  ShowAdditionalParam=off  OutDataTypeStr=uint8
  check TxB0 : Subsystem  TreatAsAtomicUnit=on
  load Tx data : Subsystem  TreatAsAtomicUnit=on
  send TxB0 : Subsystem  TreatAsAtomicUnit=on
  Out : Outport
  CAN_Transmitted : Outport  Port=2
  wires:
  In/1 -> load Tx data/1(In1)
  load Tx data/1(Out1) -> send TxB0/1(In1)
  send TxB0/1(Out1) -> check TxB0/1(In1)
  check TxB0/1(Out1) -> Out/1
  check TxB0/2(CANTx_Transmit) -> CAN_Transmitted/1
  CAN_ext/1 -> load Tx data/2(CAN_ext)
  CAN_id/1 -> load Tx data/3(CAN_id)
  CAN_dlc/1 -> load Tx data/4(CAN_dlc)
  CAN_data/1 -> load Tx data/5(CAN_data)

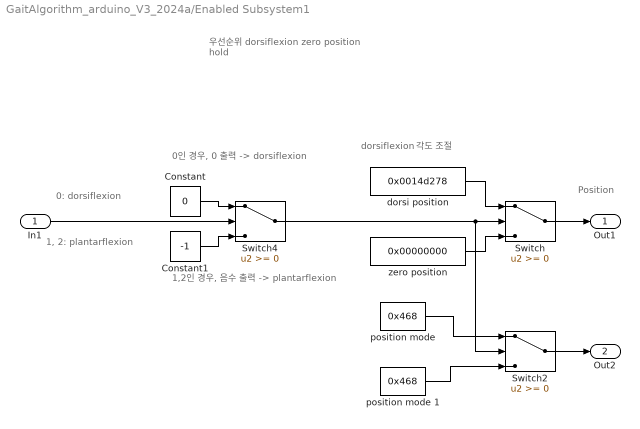
== system GaitAlgorithm_arduino_V3_2024a/Enabled Subsystem1 ==
  note: dorsiflexion 각도 조절
  note: 우선순위
      | dorsiflexion
      | zero position
      | hold
  note: Position
  note: 0: dorsiflexion
  note: 1, 2: plantarflexion
  note: 1,2인 경우, 음수 출력 -> plantarflexion
  note: 0인 경우, 0 출력 -> dorsiflexion
  In1 : Inport
  Constant : Constant  Value=0
  Constant1 : Constant  Value=-1
  Switch : Switch  OutDataTypeStr=uint32  SaturateOnIntegerOverflow=off  InputSameDT=off
  Switch2 : Switch  OutDataTypeStr=uint32  SaturateOnIntegerOverflow=off  InputSameDT=off
  Switch4 : Switch  SaturateOnIntegerOverflow=off  InputSameDT=off
  dorsi position : Constant  Value=0x0014d278
  "position mode " : Constant  Value=0x468
  position mode 1 : Constant  Value=0x468
  zero position : Constant  Value=0x00000000
  Out1 : Outport
  Out2 : Outport  Port=2
  wires:
  Switch/1 -> Out1/1
  dorsi position/1 -> Switch/1
  "position mode "/1 -> Switch2/1
  In1/1 -> Switch4/2
  Constant/1 -> Switch4/1
  Constant1/1 -> Switch4/3
  zero position/1 -> Switch/3
  Switch2/1 -> Out2/1
  position mode 1/1 -> Switch2/3
  Switch4/1 -> Switch2/2, Switch/2

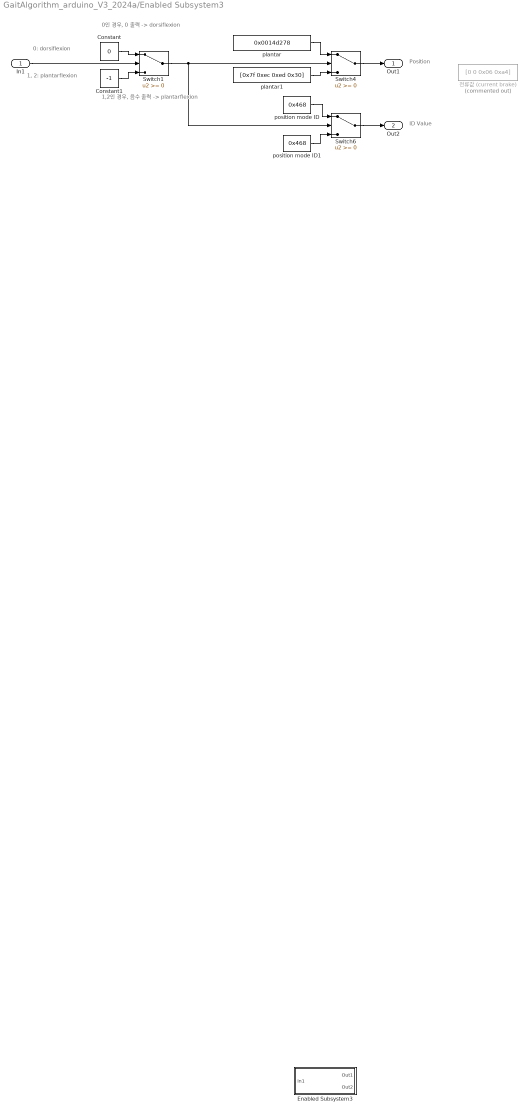
== system GaitAlgorithm_arduino_V3_2024a/Enabled Subsystem3 ==
  note: ID Value
  note: Position
  note: 1,2인 경우, 음수 출력 -> plantarflexion
  note: 0인 경우, 0 출력 -> dorsiflexion
  note: 1, 2: plantarflexion
  note: 0: dorsiflexion
  In1 : Inport
  Constant : Constant  Value=0
  Constant1 : Constant  Value=-1
  Enabled Subsystem3 : Subsystem  TreatAsAtomicUnit=on
  Switch1 : Switch  SaturateOnIntegerOverflow=off  InputSameDT=off
  Switch4 : Switch  OutDataTypeStr=uint32  SaturateOnIntegerOverflow=off  InputSameDT=off
  Switch6 : Switch  OutDataTypeStr=uint32  SaturateOnIntegerOverflow=off  InputSameDT=off
  plantar : Constant  Value=0x0014d278
  plantar1 : Constant  Value=[0x7f 0xec 0xed 0x30]
  position mode ID : Constant  Value=0x468
  position mode ID1 : Constant  Value=0x468
  전류값 (current brake) : Constant  Commented=on  Value=[0 0 0x06 0xa4]  OutDataTypeStr=uint8
  Out1 : Outport
  Out2 : Outport  Port=2
  wires:
  Switch6/1 -> Out2/1
  plantar/1 -> Switch4/1
  position mode ID/1 -> Switch6/1
  position mode ID1/1 -> Switch6/3
  Switch4/1 -> Out1/1
  In1/1 -> Switch1/2
  Constant/1 -> Switch1/1
  Constant1/1 -> Switch1/3
  Switch1/1 -> Switch6/2, Switch4/2
  plantar1/1 -> Switch4/3

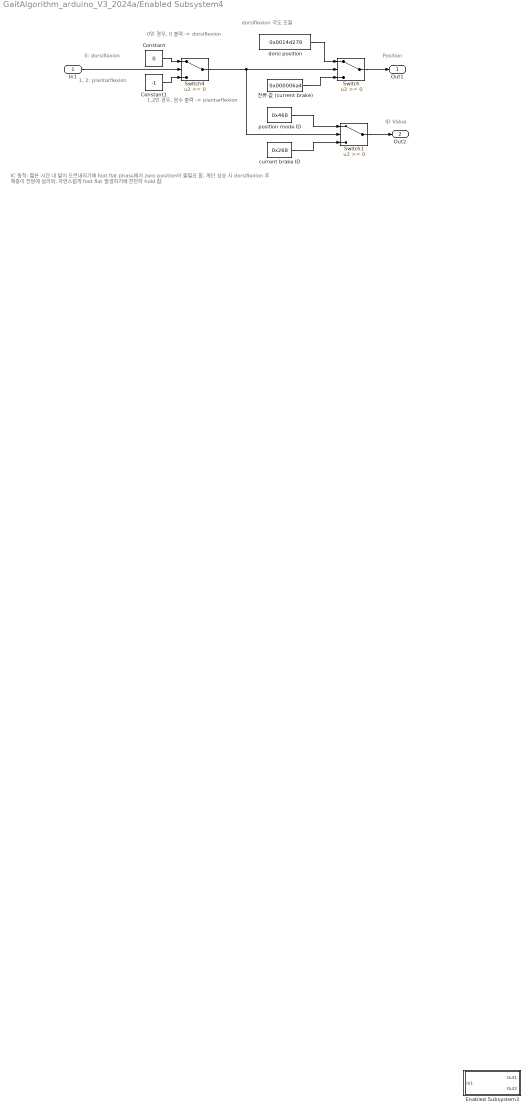
== system GaitAlgorithm_arduino_V3_2024a/Enabled Subsystem4 ==
  note: ID Value
  note: Position
  note: dorsiflexion 각도 조절
  note: IC 동작: 짧은 시간 내 발이 오르내리기에 foot flat phase에서 zero position이 불필요 함.
      | 계단 상승 시 dorsiflexion 후 체중이 전방에 실리며, 자연스럽게 foot flat 발생하기에 천천히 hold 함.
  note: 1,2인 경우, 음수 출력 -> plantarflexion
  note: 0인 경우, 0 출력 -> dorsiflexion
  note: 1, 2: plantarflexion
  note: 0: dorsiflexion
  In1 : Inport
  " 전류 값 (current brake)" : Constant  Value=0x000006a4
  Constant : Constant  Value=0
  Constant1 : Constant  Value=-1
  Enabled Subsystem3 : Subsystem  TreatAsAtomicUnit=on
  Switch : Switch  OutDataTypeStr=uint32  SaturateOnIntegerOverflow=off  InputSameDT=off
  Switch1 : Switch  OutDataTypeStr=uint32  SaturateOnIntegerOverflow=off  InputSameDT=off
  Switch4 : Switch  SaturateOnIntegerOverflow=off  InputSameDT=off
  current brake ID : Constant  Value=0x268
  dorsi position : Constant  Value=0x0014d278
  position mode ID : Constant  Value=0x468
  Out1 : Outport
  Out2 : Outport  Port=2
  wires:
  Switch/1 -> Out1/1
  Switch1/1 -> Out2/1
  dorsi position/1 -> Switch/1
  " 전류 값 (current brake)"/1 -> Switch/3
  position mode ID/1 -> Switch1/1
  current brake ID/1 -> Switch1/3
  In1/1 -> Switch4/2
  Constant/1 -> Switch4/1
  Switch4/1 -> Switch1/2, Switch/2
  Constant1/1 -> Switch4/3

== system GaitAlgorithm_arduino_V3_2024a/Subsystem ==
  note: UDP signal
      | : 1,2,3
  note: LG - position
  note: IC - position
  note: DC - position
  note: etc
  In1 : Inport
  In2 : Inport  Port=2
  In3 : Inport  Port=3
  In5 : Inport  Port=4
  In6 : Inport  Port=5
  Switch1 : Switch  Criteria=u2 > Threshold  Threshold=1  SaturateOnIntegerOverflow=off  InputSameDT=off
  Switch3 : Switch  Criteria=u2 > Threshold  SaturateOnIntegerOverflow=off  InputSameDT=off
  Switch4 : Switch  SaturateOnIntegerOverflow=off  InputSameDT=off
  Out1 : Outport
  wires:
  In2/1 -> Switch1/3
  In3/1 -> Switch1/1
  Switch1/1 -> Switch3/1
  Switch3/1 -> Out1/1
  In5/1 -> Switch4/2, Switch3/2, Switch1/2
  Switch4/1 -> Switch3/3
  In1/1 -> Switch4/1
  In6/1 -> Switch4/3

== system GaitAlgorithm_arduino_V3_2024a/Subsystem1 ==
  note: LG - position
  note: DC - position
  note: UDP signal
      | : 1,2,3
  note: IC - position
  In1 : Inport
  In2 : Inport  Port=2
  In3 : Inport  Port=3
  In5 : Inport  Port=4
  In6 : Inport  Port=5
  Switch1 : Switch  Criteria=u2 > Threshold  Threshold=1  SaturateOnIntegerOverflow=off  InputSameDT=off
  Switch3 : Switch  Criteria=u2 > Threshold  SaturateOnIntegerOverflow=off  InputSameDT=off
  Switch4 : Switch  SaturateOnIntegerOverflow=off  InputSameDT=off
  Out1 : Outport
  wires:
  In2/1 -> Switch1/3
  In3/1 -> Switch1/1
  Switch1/1 -> Switch3/1
  Switch3/1 -> Out1/1
  In5/1 -> Switch1/2, Switch3/2, Switch4/2
  Switch4/1 -> Switch3/3
  In1/1 -> Switch4/1
  In6/1 -> Switch4/3

== system GaitAlgorithm_arduino_V3_2024a/CANbegin/setup ==
  Enable : EnablePort
  CNF1 : Constant  Value=address2A  OutDataTypeStr=uint8
  CNF2 : Constant  Value=address29  OutDataTypeStr=uint8
  CNF3 : Constant  Value=address28  OutDataTypeStr=uint8
  Ground : Ground
  Terminator : Terminator
  changeCANmode(config) : Subsystem  TreatAsAtomicUnit=on
  changeCANmode(normal) : Subsystem  TreatAsAtomicUnit=on
  mcp2515_reset : Subsystem  TreatAsAtomicUnit=on
  setCANRxBuffer : Subsystem  TreatAsAtomicUnit=on
  setCANspeed : Subsystem  TreatAsAtomicUnit=on
  wires:
  CNF3/1 -> setCANspeed/4(CNF3)
  CNF2/1 -> setCANspeed/3(CNF2)
  CNF1/1 -> setCANspeed/2(CNF1)
  mcp2515_reset/1(Out) -> changeCANmode(config)/1(In)
  changeCANmode(config)/1(Out) -> setCANspeed/1(In)
  setCANspeed/1(Out) -> setCANRxBuffer/1(In)
  setCANRxBuffer/1(Out) -> changeCANmode(normal)/1(In)
  Ground/1 -> mcp2515_reset/1(In)
  changeCANmode(normal)/1(Out) -> Terminator/1

== system GaitAlgorithm_arduino_V3_2024a/CANreceive/checkRxMsgStatus ==
  RX_STATUS : Inport
  Bitmask_RxBn : simulink/Logic and Bit Operations/Bitwise Operator  logicop=AND  UseBitMask=on  BitMask=bin2dec('11000000')  BitMaskRealWorld=Stored Integer
  CAN_NOMSG : Constant  Value=-1  OutDataTypeStr=int8
  CAN_OK : Constant  OutDataTypeStr=int8
  Switch : Switch  Criteria=u2 > Threshold  SaturateOnIntegerOverflow=off  InputSameDT=off
  CANRx_Received : Outport
  wires:
  RX_STATUS/1 -> Bitmask_RxBn/1
  CAN_OK/1 -> Switch/1
  CAN_NOMSG/1 -> Switch/3
  Switch/1 -> CANRx_Received/1
  Bitmask_RxBn/1 -> Switch/2

== system GaitAlgorithm_arduino_V3_2024a/CANreceive/mcp2515_read_RX_STATUS ==
  In : Inport
  Constant : Constant  Value=0  OutDataTypeStr=uint8
  MCP_RX_STATUS : Constant  Value=hex2dec('B0')  OutDataTypeStr=uint8
  SPI driver : mcp2515lib/CAN application/mcp2515 driver/SPI driver  SystemSampleTime=-1  VariantActivationTime=update diagram  AllowFlexibleInterface=on  Latency=0  AutoFrameSizeCalculation=off
      settings: SourceProductName=CAN device driver for mcp2515
  Selector : Selector  IndexMode=Zero-based  InputPortWidth=2  IndexOptions=Index vector (dialog)  Indices=1  OutputSizes=1
  Vector Concatenate : Concatenate
  Out : Outport
  RX_STATUS : Outport  Port=2
  wires:
  In/1 -> Out/1
  Constant/1 -> Vector Concatenate/2
  SPI driver/1 -> Selector/1
  Selector/1 -> RX_STATUS/1
  MCP_RX_STATUS/1 -> Vector Concatenate/1
  Vector Concatenate/1 -> SPI driver/1
